simulink model "new_analog_loopback_q4_2000hz_bettersampled"  (R2017a)
settings: Solver=FixedStepDiscrete  StartTime=0.0  StopTime=inf  FixedStep=0.00005  RelTol=1e-3  EnableMultiTasking=on
StopFcn:
  | run('graph_2000hz_bettersampled.m');
libraries: xpcquanserlib x2, slrtlib x2
settings Model: SimulationMode=external  Creator=Venkatraman  LastModifiedBy=awlloyd
settings SolverCC: EnableConcurrentExecution=on
settings DataIOCC: LimitDataPoints=on  SaveFormat=Array  LoggingToFile=on
settings OptimizationCC: BlockReduction=off  OptimizeBlockIOStorage=off  BufferReuse=off  GlobalBufferReuse=off  ExpressionFolding=off  LocalBlockOutputs=off  LifeSpan=inf
settings DebuggingCC: SolverPrmCheckMsg=warning  SFUnexpectedBacktrackingDiag=warning  SFNoUnconditionalDefaultTransitionDiag=warning  SFExecutionAtInitializationDiag=none
settings HardwareCC: ProdBitPerPointer=32  ProdBitPerSizeT=32  ProdBitPerPtrDiffT=32  ProdLargestAtomicFloat=None  ProdWordSize=32  ProdLongLongMode=on  ProdHWDeviceType=Generic->32-bit x86 compatible  TargetBitPerPointer=64  TargetBitPerSizeT=64  TargetBitPerPtrDiffT=64  TargetLongLongMode=on  TargetIntDivRoundTo=Zero  TargetEndianess=LittleEndian  TargetWordSize=64  TargetHWDeviceType=MATLAB Host
settings ModelReferenceCC: PropagateSignalLabelsOutOfModel=off
settings RTWCC: SystemTargetFile=slrt.tlc  TemplateMakefile=slrt_default_tmf  Description=Simulink Real-Time  RTWVerbose=off  RTWCompilerOptimization=on
settings SimulinkRealTimeCC: GeneratePreprocessorConditionals=Disable all
settings ConfigComp: CovMetricSettings=dw  CovHtmlReporting=on  CovSaveCumulativeToWorkspaceVar=on  CovSaveSingleToWorkspaceVar=on  CovExternalEMLEnable=off  CovSFcnEnable=off

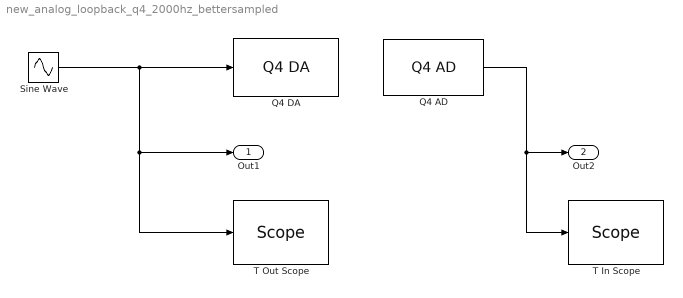
== system new_analog_loopback_q4_2000hz_bettersampled ==
  Q4 AD : xpcquanserlib/A//D/Q4 AD  channel=[2]  sampleTime=0.00005  slot=-1
      settings: SourceProductName=Simulink Real-Time  SourceProductBaseCode=XP
  "Q4 DA " : xpcquanserlib/D//A/Q4 DA   channel=[1]  range=[-5]  simul=off  reset=[1]  initValue=[0]  sampleTime=.00005  slot=-1
      settings: SourceProductName=Simulink Real-Time  SourceProductBaseCode=XP
  Sine Wave : Sin  Frequency=2*pi*2000  SampleTime=0
  T In Scope : slrtlib/Displays and Logging/Scope   scopeno=2  scopetype=Target  autostart=on  viewmode=Graphical rolling  formatstr='%15.6f'  grid=on  ylimits=[-1,1]  nosamples=250  noprepostsamples=0  interleave=1  triggermode=FreeRun  triggersignal=1  trigsignalfromport=off  triggerlevel=0.0  triggerslope=Either  triggerscope=1  triggersample=0  filename=data.dat  mode=Lazy  writesize=512  autorestart=off  dynamicfilemode=off  maxwritefilesize=512*1024^2
  T Out Scope : slrtlib/Displays and Logging/Scope   scopeno=1  scopetype=Target  autostart=on  viewmode=Graphical rolling  formatstr='%15.6f'  grid=on  ylimits=[-1,1]  nosamples=250  noprepostsamples=0  interleave=1  triggermode=FreeRun  triggersignal=1  trigsignalfromport=off  triggerlevel=0.0  triggerslope=Either  triggerscope=1  triggersample=0  filename=data.dat  mode=Lazy  writesize=512  autorestart=off  dynamicfilemode=off  maxwritefilesize=512*1024^2
  Out1 : Outport
  Out2 : Outport  Port=2
  wires:
  Q4 AD/1 -> T In Scope/1, Out2/1
  Sine Wave/1 -> "Q4 DA "/1, T Out Scope/1, Out1/1
